simulink model "Lab_3_BD1"  (R2024a)
settings: Solver=VariableStepAuto  StartTime=0.0  StopTime=20  RelTol=1e-3
values from neighbouring files (symbols this model uses):
  G1_den = [1 0 0]    [Lab_3_BD1.m]    (also in Laboratory_3_No_2.m)
  G1_num = [1]    [Lab_3_BD1.m]    (also in Laboratory_3_No_2.m)
  G2_den = [1 1]    [Lab_3_BD1.m]    (also in Laboratory_3_No_2.m)
  G2_num = [1]    [Lab_3_BD1.m]    (also in Laboratory_3_No_2.m)
  G3_den = [1 0]    [Lab_3_BD1.m]    (also in Laboratory_3_No_2.m)
  G3_num = [1]    [Lab_3_BD1.m]    (also in Laboratory_3_No_2.m)
  H1_den = [1 0]    [Lab_3_BD1.m]    (also in Laboratory_3_No_2.m)
  H1_num = [1]    [Lab_3_BD1.m]    (also in Laboratory_3_No_2.m)
  H2_den = [1 -1]    [Lab_3_BD1.m]    (also in Laboratory_3_No_2.m)
  H2_num = [1]    [Lab_3_BD1.m]    (also in Laboratory_3_No_2.m)
  H3_den = [1 -2]    [Lab_3_BD1.m]    (also in Laboratory_3_No_2.m)
  H3_num = [1]    [Lab_3_BD1.m]    (also in Laboratory_3_No_2.m)
settings Model: LastModifiedBy=Sydney Ruoj

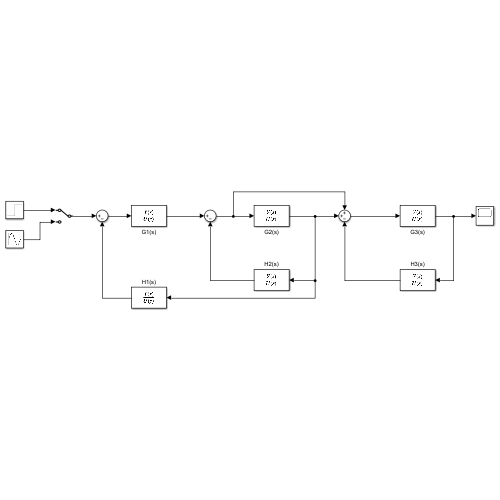
[thumbnail: Simulink's stored preview of the top-level diagram]
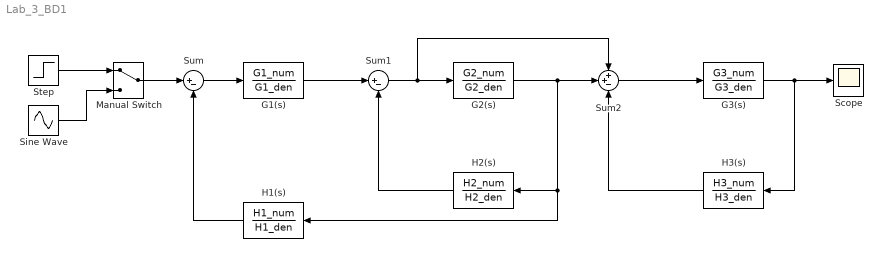
== system Lab_3_BD1 ==
  G1(s) : TransferFcn  Numerator=G1_num  Denominator=G1_den
  G2(s) : TransferFcn  Numerator=G2_num  Denominator=G2_den
  G3(s) : TransferFcn  Numerator=G3_num  Denominator=G3_den
  H1(s) : TransferFcn  Numerator=H1_num  Denominator=H1_den
  H2(s) : TransferFcn  Numerator=H2_num  Denominator=H2_den
  H3(s) : TransferFcn  Numerator=H3_num  Denominator=H3_den
  Manual Switch : ManualSwitch
  Scope : Scope
  Sine Wave : Sin  SampleTime=0
  Step : Step  Time=0  SampleTime=0
  Sum : Sum  Inputs=|+-
  Sum1 : Sum  Inputs=|+-
  Sum2 : Sum  Inputs=++-
  wires:
  Sum/1 -> G1(s)/1
  G1(s)/1 -> Sum1/1
  Sum1/1 -> Sum2/1, G2(s)/1
  G2(s)/1 -> H1(s)/1, H2(s)/1, Sum2/2
  Sum2/1 -> G3(s)/1
  G3(s)/1 -> H3(s)/1, Scope/1
  H3(s)/1 -> Sum2/3
  H2(s)/1 -> Sum1/2
  H1(s)/1 -> Sum/2
  Manual Switch/1 -> Sum/1
  Step/1 -> Manual Switch/1
  Sine Wave/1 -> Manual Switch/2
